simulink model "simulinkdynamics"  (R2020a)
settings: Solver=FixedStepAuto  StartTime=0.0  StopTime=20  FixedStep=0.0001  RelTol=1e-3
values from neighbouring files (symbols this model uses):
  K = 0.0879    [dinamica.m]
undefined symbols (not defined in the file or in its folder): Nbar
libraries: simulink x2
settings Model: Creator=USUARIO  LastModifiedBy=charlie
settings DataIOCC: ReturnWorkspaceOutputs=off
settings DebuggingCC: ArithmeticOperatorsInVariantConditions=warning
settings SFSimCC: CustomCodeUndefinedFunction=UseInterfaceOnly

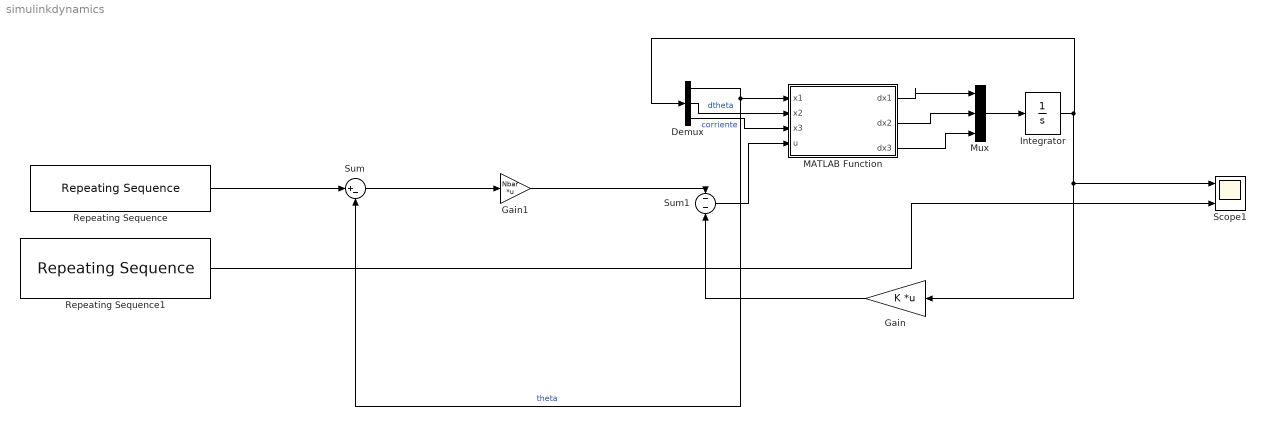
== system simulinkdynamics ==
  Demux : Demux  Outputs=3
  Gain : Gain  Gain=K  Multiplication=Matrix(K*u) (u vector)
  Gain1 : Gain  Gain=Nbar  Multiplication=Matrix(K*u) (u vector)
  Integrator : Integrator
  MATLAB Function : MATLAB Function  TreatAsAtomicUnit=on
  Mux : Mux  Inputs=3
  Repeating Sequence : simulink/Sources/Repeating Sequence  rep_seq_t=tiempo  rep_seq_y=pos_norm
  Repeating Sequence1 : simulink/Sources/Repeating Sequence  rep_seq_t=tiempo  rep_seq_y=vel_norm
  Scope1 : Scope  NumInputPorts=3
  Sum : Sum  Inputs=|+-
  Sum1 : Sum  Inputs=--
  wires:
  MATLAB Function/1(dx1) -> Mux/1
  MATLAB Function/2(dx2) -> Mux/2
  MATLAB Function/3(dx3) -> Mux/3
  Mux/1 -> Integrator/1
  Demux/1 -> MATLAB Function/1(x1), Sum/2  "theta"
  Demux/2 -> MATLAB Function/2(x2)  "dtheta"
  Demux/3 -> MATLAB Function/3(x3)  "corriente"
  Sum1/1 -> MATLAB Function/4(u)
  Gain/1 -> Sum1/2
  Sum/1 -> Gain1/1
  Gain1/1 -> Sum1/1
  Repeating Sequence1/1 -> Scope1/3
  Integrator/1 -> Scope1/1, Gain/1, Demux/1
  Repeating Sequence/1 -> Sum/1

== matlab function simulinkdynamics/MATLAB Function ==
  data: x1 input; x2 input; x3 input; u input; dx1 output; dx2 output; dx3 output
function [dx1,dx2,dx3] = dinamica(x1,x2,x3,u)
%UNTITLED2 Summary of this function goes here
%   Detailed explanation goes here
G = 9.8;
B = 0.01;
J = 3;
L = 0.001;
R = 0.1;
K = 0.0879;
r = 2;
dx1 = x2; 
dx2 = sin(x1) * G / (J*r)  - x2* B / (J*r) + K * x3 ;
dx3 = - x2* K/ L - x3 * R / L + u / L;
end
